simulink model "simulink"  (R2015a)
settings: Solver=ode45  StartTime=0.0  StopTime=2  RelTol=1e-3
values from neighbouring files (symbols this model uses):
  C = sistema_adpt_d.C    [main.m]
  G = sistema_adpt_d.A    [main.m]
  H = sistema_adpt_d.B    [main.m]
  K1 = K(3)    [main.m]
  K2 = [K(1) K(2)]    [main.m]
  L = L'    [main.m]
  T = T*11    (= 0.011)    [main.m]
undefined symbols (not defined in the file or in its folder): Beq, Eff_g, Eff_m, IMAX_AMP, Jm, Kg, Km, Kt, M, r_mp, Rm
settings Model: Creator=Pedro Pereira  LastModifiedBy=Pedro Pereira

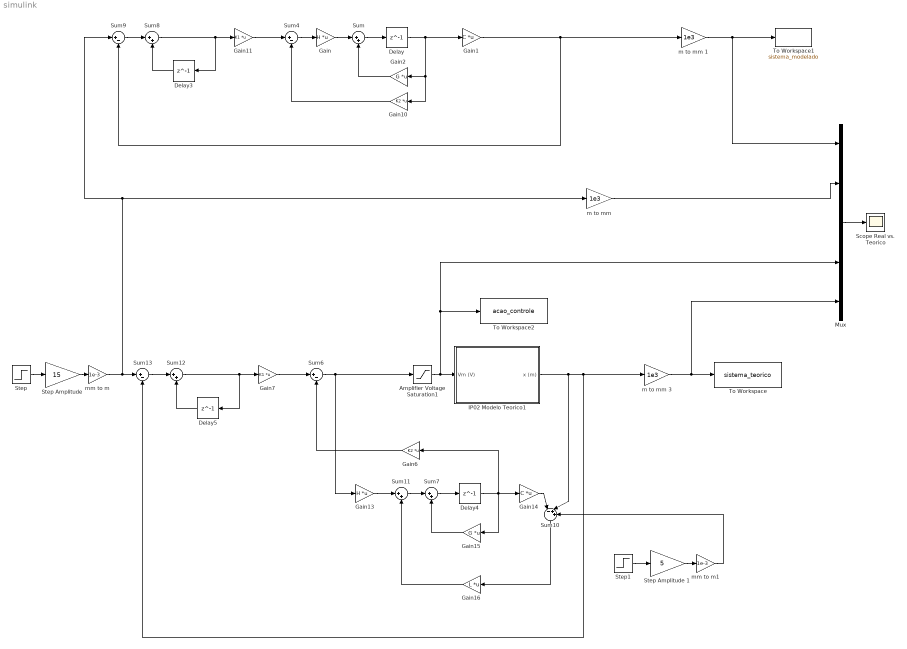
== system simulink ==
  Amplifier Voltage Saturation1 : Saturate  UpperLimit=8  LowerLimit=-8
  Delay{,3..5} (4 alike) : Delay  DelayLength=1  SampleTime=T
  Gain : Gain  Gain=H  Multiplication=Matrix(K*u)
  Gain1 : Gain  Gain=C  Multiplication=Matrix(K*u)
  Gain10 : Gain  Gain=K2  Multiplication=Matrix(K*u)
  Gain11 : Gain  Gain=K1  Multiplication=Matrix(K*u)
  Gain13 : Gain  Gain=H  Multiplication=Matrix(K*u)
  Gain14 : Gain  Gain=C  Multiplication=Matrix(K*u)
  Gain15 : Gain  Gain=G  Multiplication=Matrix(K*u)
  Gain16 : Gain  Gain=L  Multiplication=Matrix(K*u)
  Gain2 : Gain  Gain=G  Multiplication=Matrix(K*u)
  Gain6 : Gain  Gain=K2  Multiplication=Matrix(K*u)
  Gain7 : Gain  Gain=K1  Multiplication=Matrix(K*u)
  IP02 Modelo Teorico1 : Subsystem
  Mux : Mux  Inputs=5
  Scope Real vs. Teorico : Scope
      settings: TickLabels=on  TimeRange=5  YMin=-11  YMax=11  SaveName=x  MaxDataPoints=2500
  Step : Step  Time=0  SampleTime=T
  "Step Amplitude " : Gain  Gain=15  SaturateOnIntegerOverflow=on  OutDataTypeStr=Inherit: Same as input  ParamDataTypeStr=Inherit: Same as input
  Step Amplitude 1 : Gain  Gain=5  SaturateOnIntegerOverflow=on  OutDataTypeStr=Inherit: Same as input  ParamDataTypeStr=Inherit: Same as input
  Step1 : Step  Time=0  SampleTime=T
  Sum{,7..8,11..12} (5 alike) : Sum  Inputs=|++
  Sum10 : Sum  Inputs=|-++
  Sum{4,6,9,13} (4 alike) : Sum  Inputs=|+-
  To Workspace : ToWorkspace  VariableName=sistema_teorico  SaveFormat=Timeseries  SampleTime=-1
  To Workspace1 : ToWorkspace  VariableName=sistema_modelado  SaveFormat=Timeseries  SampleTime=-1
  To Workspace2 : ToWorkspace  VariableName=acao_controle  SaveFormat=Timeseries  SampleTime=-1
  "m to mm " : Gain  Gain=1e3  SaturateOnIntegerOverflow=on  OutDataTypeStr=Inherit: Same as input  ParamDataTypeStr=Inherit: Same as input
  m to mm 1 : Gain  Gain=1e3  SaturateOnIntegerOverflow=on  OutDataTypeStr=Inherit: Same as input  ParamDataTypeStr=Inherit: Same as input
  m to mm 3 : Gain  Gain=1e3  SaturateOnIntegerOverflow=on  OutDataTypeStr=Inherit: Same as input  ParamDataTypeStr=Inherit: Same as input
  mm to m : Gain  Gain=1e-3
  mm to m1 : Gain  Gain=1e-3
  wires:
  Mux/1 -> Scope Real vs. Teorico/1
  Step/1 -> "Step Amplitude "/1
  "m to mm "/1 -> Mux/2
  Gain/1 -> Sum/1
  Sum/1 -> Delay/1
  Delay/1 -> Gain10/1, Gain2/1, Gain1/1
  Gain2/1 -> Sum/2
  m to mm 1/1 -> To Workspace1/1, Mux/1
  Sum4/1 -> Gain/1
  Gain10/1 -> Sum4/2
  Gain11/1 -> Sum4/1
  Sum8/1 -> Delay3/1, Gain11/1
  Delay3/1 -> Sum8/2
  Sum9/1 -> Sum8/1
  Gain1/1 -> Sum9/2, m to mm 1/1
  Sum6/1 -> Amplifier Voltage Saturation1/1, Gain13/1
  Sum7/1 -> Delay4/1
  Delay4/1 -> Gain6/1, Gain15/1, Gain14/1
  Gain15/1 -> Sum7/2
  Gain14/1 -> Sum10/1
  Sum10/1 -> Gain16/1
  Sum11/1 -> Sum7/1
  Gain13/1 -> Sum11/1
  Gain16/1 -> Sum11/2
  Gain7/1 -> Sum6/1
  Sum12/1 -> Delay5/1, Gain7/1
  Delay5/1 -> Sum12/2
  Sum13/1 -> Sum12/1
  mm to m/1 -> Sum13/1, "m to mm "/1, Sum9/1
  Amplifier Voltage Saturation1/1 -> To Workspace2/1, Mux/4, IP02 Modelo Teorico1/1(Vm (V))
  IP02 Modelo Teorico1/1(x (m)) -> Sum10/2, Sum13/2, m to mm 3/1
  m to mm 3/1 -> Mux/5, To Workspace/1
  "Step Amplitude "/1 -> mm to m/1
  Step1/1 -> Step Amplitude 1/1
  Step Amplitude 1/1 -> mm to m1/1
  Gain6/1 -> Sum6/2
  mm to m1/1 -> Sum10/3

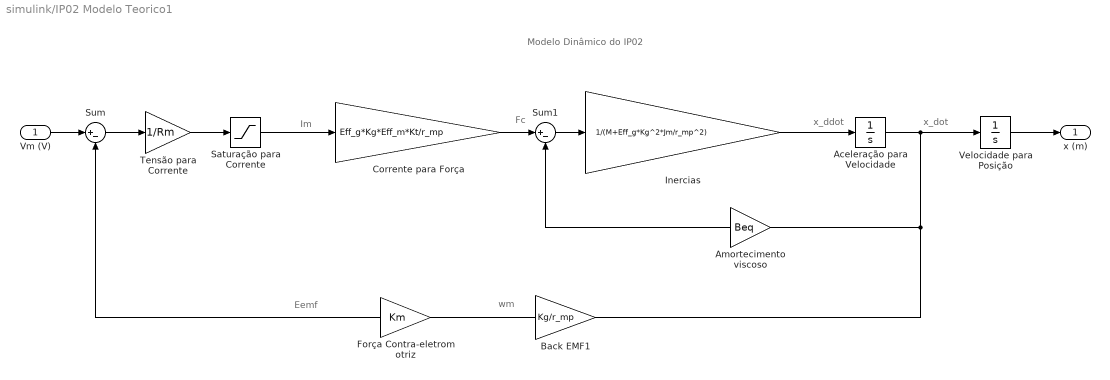
== system simulink/IP02 Modelo Teorico1 ==
  note: Modelo Dinâmico do IP02
  note: Fc
  note: Im
  note: Eemf
  note: wm
  note: x_dot
  note: x_ddot
  Vm (V) : Inport
  Aceleração para Velocidade : Integrator
  Amortecimento viscoso : Gain  Gain=Beq  SaturateOnIntegerOverflow=on  OutDataTypeStr=Inherit: Same as input  ParamDataTypeStr=Inherit: Same as input
  Back EMF1 : Gain  Gain=Kg/r_mp  SaturateOnIntegerOverflow=on  OutDataTypeStr=Inherit: Same as input  ParamDataTypeStr=Inherit: Same as input
  Corrente para Força : Gain  Gain=Eff_g*Kg*Eff_m*Kt/r_mp  SaturateOnIntegerOverflow=on  OutDataTypeStr=Inherit: Same as input  ParamDataTypeStr=Inherit: Same as input
  Força Contra-eletromotriz : Gain  Gain=Km  SaturateOnIntegerOverflow=on  OutDataTypeStr=Inherit: Same as input  ParamDataTypeStr=Inherit: Same as input
  Inercias : Gain  Gain=1/(M+Eff_g*Kg^2*Jm/r_mp^2)  SaturateOnIntegerOverflow=on  OutDataTypeStr=Inherit: Same as input  ParamDataTypeStr=Inherit: Same as input
  Saturação para Corrente : Saturate  UpperLimit=IMAX_AMP  LowerLimit=- IMAX_AMP
  Sum : Sum  Inputs=|+-  SaturateOnIntegerOverflow=on  InputSameDT=on  OutDataTypeStr=Inherit: Same as first input
  Sum1 : Sum  Inputs=|+-  SaturateOnIntegerOverflow=on  InputSameDT=on  OutDataTypeStr=Inherit: Same as first input
  Tensão para Corrente : Gain  Gain=1/Rm  SaturateOnIntegerOverflow=on  OutDataTypeStr=Inherit: Same as input  ParamDataTypeStr=Inherit: Same as input
  Velocidade para Posição : Integrator
  x (m) : Outport
  wires:
  Sum/1 -> Tensão para Corrente/1
  Inercias/1 -> Aceleração para Velocidade/1
  Sum1/1 -> Inercias/1
  Tensão para Corrente/1 -> Saturação para Corrente/1
  Aceleração para Velocidade/1 -> Velocidade para Posição/1, Back EMF1/1, Amortecimento viscoso/1
  Back EMF1/1 -> Força Contra-eletromotriz/1
  Saturação para Corrente/1 -> Corrente para Força/1
  Vm (V)/1 -> Sum/1
  Velocidade para Posição/1 -> x (m)/1
  Corrente para Força/1 -> Sum1/1
  Amortecimento viscoso/1 -> Sum1/2
  Força Contra-eletromotriz/1 -> Sum/2
